simulink model "Ex3"  (R2024b)
settings: Solver=VariableStepAuto  StartTime=0.0  StopTime=1000  FixedStep=0.1  MaxStep=0.01  RelTol=1e-3
undefined symbols (not defined in the file): Ion, Lithium
libraries: spsBatteryLib x1, spsControlledCurrentSourceLib x1, spsDCMachineLib x1, sps_lib x1
settings Model: Creator=balaj  LastModifiedBy=balaj

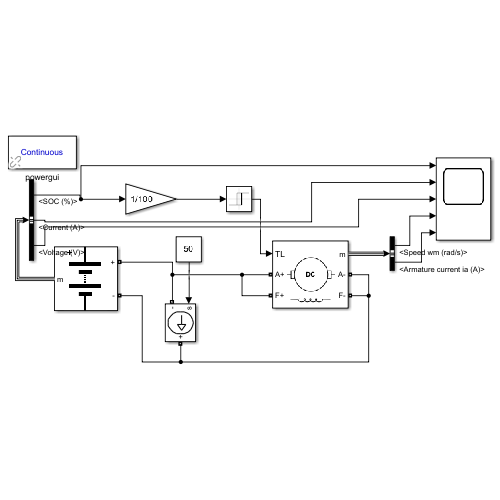
[thumbnail: Simulink's stored preview of the top-level diagram]
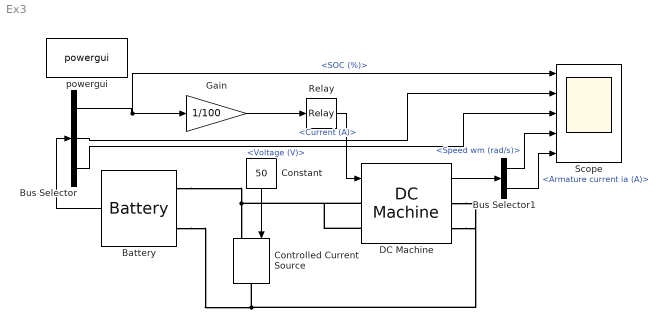
== system Ex3 ==
  Battery : spsBatteryLib/Battery  BatType=Lithium-Ion  NomV=200  NomQ=6.5  SOC=100  Batt_Tr=30  PresetModel=on  MaxQ=6.5  MinV=150  FullV=232.7974  Dis_rate=2.8261  R=0.30769  Normal_OP=5.8783  expZone="[216.0772     0.3193478]"
  Bus Selector : BusSelector  OutputSignals=SOC (%),Current (A),Voltage (V)
  Bus Selector1 : BusSelector  OutputSignals=Speed wm (rad/s),Armature current ia (A)
  Constant : Constant  Value=50
  Controlled Current Source : spsControlledCurrentSourceLib/Controlled Current Source  Initialize=on  Source_Type=AC  Amplitude=0  Phase=0  Frequency=0  Measurements=None
  DC Machine : spsDCMachineLib/DC Machine  PresetModel=No  MechanicalLoad=Torque TL  FieldType=Wound  ShowDetailedParameters=on  MeasurementBus=off  RLa="[ 0.6  0.012]"  RLf="[ 240  120]"  Laf=1.8  MachineConstant=Torque constant (N.m/A)  Ke=1.8  Kt=1.8  J=1  Bm=0  Tf=0  w0=1  Ifinit=0  TsPowergui=0  TsBlock=-1
  Gain : Gain  Gain=1/100
  Relay : Relay  OnSwitchValue=0.8  OffSwitchValue=0.4  OffOutputValue=-200
  Scope : Scope  NumInputPorts=5
  powergui : sps_lib/powergui  Priority=1  SimulationMode=Continuous  SampleTime=50e-6  frequency=60  Iterations=50  frequencyindice=0  Pbase=100e6  ErrMax=1e-4  UnitsV=kV  UnitsW=MW  buscounter=0  FunctionMessages=off  echomessages=off  EnableUseOfTLC=off  CurrentSourceSwitches=off  DisableSnubberDevices=off  DisableRonSwitches=off  DisableVfSwitches=off  DisplayEquations=off  AutomaticDiscreteSolvers=off  SolverType=Tustin/Backward Euler (TBE)  Interpol=off  ExternalGateDelay=off  methode=off  Ts=100  x0status=blocks  SPID=on  SwTol=0  HookPort=off  NonlinearTolerance=1e-4  nMaxIteration=100  ContinueOnMaxIteration=off  RestoreLinks=warning  ResistiveCurrentMeasurement=off  Frange=[0:2:500]  Ylog=off  Xlog=on  ShowGrid=off  save=off  variable=ZData  structure=0  ZoomFFT=off  StartTime=0.0  cycles=1  DisplayStyle=1  fundamental=60  FreqAxis=off  MaxFrequency=1000  frequencyindicesteady=1  RmsSteady=1  display=off
  wires:
  Battery/1 -> Bus Selector/1
  Bus Selector/1 -> Scope/1, Gain/1  "<SOC (%)>"
  Gain/1 -> Relay/1
  Relay/1 -> DC Machine/1
  DC Machine/1 -> Bus Selector1/1
  Bus Selector/2 -> Scope/2  "<Current (A)>"
  Bus Selector/3 -> Scope/3  "<Voltage (V)>"
  Bus Selector1/1 -> Scope/4  "<Speed wm (rad/s)>"
  Bus Selector1/2 -> Scope/5  "<Armature current ia (A)>"
  Constant/1 -> Controlled Current Source/1
  connections:
  Battery/LConn1 -- DC Machine/LConn2 -- DC Machine/LConn1 -- Controlled Current Source/LConn1
  Battery/LConn2 -- DC Machine/RConn2 -- DC Machine/RConn1 -- Controlled Current Source/RConn1
